simulink model "predator_prey"  (R2024b)
settings: Solver=VariableStepAuto  StartTime=0.0  StopTime=10.0  RelTol=1e-3
settings Model: Creator=Botló  LastModifiedBy=Botló

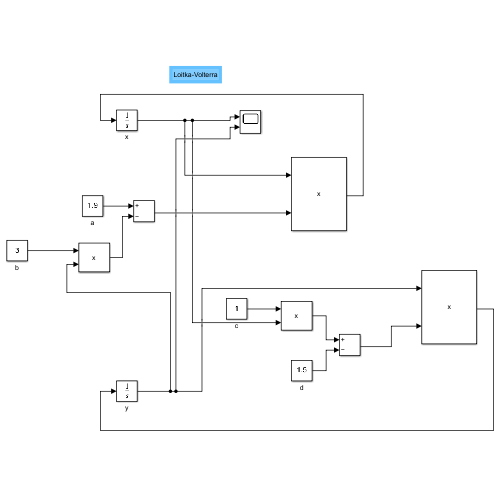
[thumbnail: Simulink's stored preview of the top-level diagram]
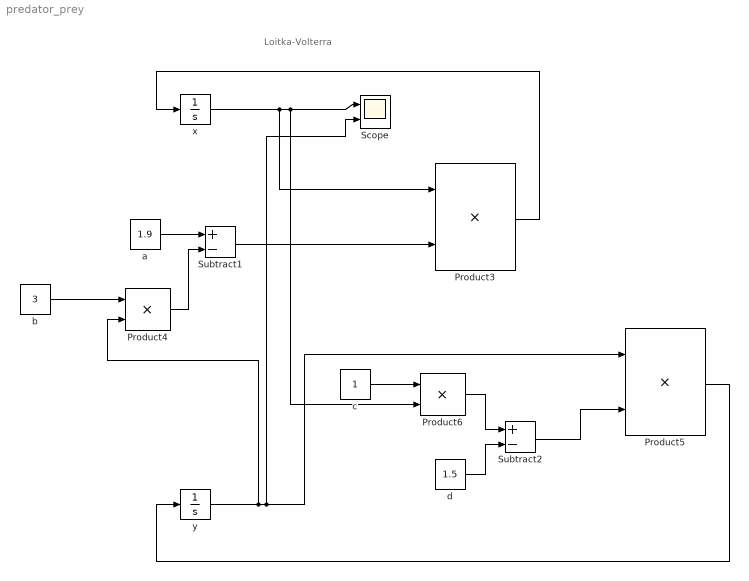
== system predator_prey ==
  note: Loitka-Volterra
  Product{3..6} (4 alike) : Product
  Scope : Scope  NumInputPorts=2
  Subtract1 : Sum  Inputs=+-
  Subtract2 : Sum  Inputs=+-
  a : Constant  Value=1.9
  b : Constant  Value=3
  c : Constant
  d : Constant  Value=1.5
  x : Integrator  InitialCondition=0.5
  y : Integrator  InitialCondition=1.5
  wires:
  b/1 -> Product4/1
  c/1 -> Product6/1
  a/1 -> Subtract1/1
  Product5/1 -> y/1
  x/1 -> Product3/1, Scope/1, Product6/2
  y/1 -> Product4/2, Product5/1, Scope/2
  Subtract2/1 -> Product5/2
  d/1 -> Subtract2/2
  Subtract1/1 -> Product3/2
  Product6/1 -> Subtract2/1
  Product4/1 -> Subtract1/2
  Product3/1 -> x/1
